simulink library "csu_rpn_ap_rpn_evaluation_lib"  (R2014b)
settings: Solver=ode45  StartTime=0.0  StopTime=10.0  RelTol=1e-3
libraries: util_info_lib x1
settings Model: Creator=escrane  LastModifiedBy=mstewart

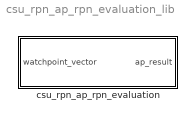
== system csu_rpn_ap_rpn_evaluation_lib ==
  csu_rpn_ap_rpn_evaluation : Subsystem  mask{rpn_equation=1 2 NOT 3 AND OR}
      mask prompts: rpn_equation "RPN Equation (numeric postfix vector)"
      mask init:
      | csu_rpn_ap_rpn_evaluation_callback(gcb, rpn_equation);
      mask Display: disp(rpn_equation);

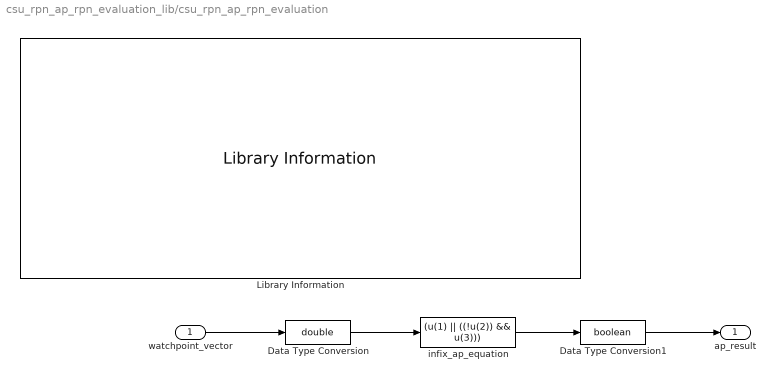
== system csu_rpn_ap_rpn_evaluation_lib/csu_rpn_ap_rpn_evaluation ==
  watchpoint_vector : Inport
  Data Type Conversion : DataTypeConversion  OutDataTypeStr=double
  Data Type Conversion1 : DataTypeConversion  OutDataTypeStr=boolean
  Library Information : util_info_lib/Library Information  owner='NONE'
  infix_ap_equation : Fcn  Expr=(u(1) || ((!u(2)) && u(3)))
  ap_result : Outport
  wires:
  Data Type Conversion/1 -> infix_ap_equation/1
  infix_ap_equation/1 -> Data Type Conversion1/1
  Data Type Conversion1/1 -> ap_result/1
  watchpoint_vector/1 -> Data Type Conversion/1
